simulink model "design_top"  (R2014a)
settings: Solver=ode45  StartTime=0.0  StopTime=10.0  RelTol=1e-3
settings Model: Creator=jan  LastModifiedBy=jan

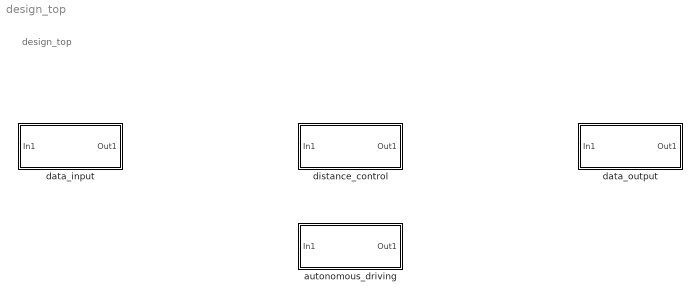
== system design_top ==
  note: design_top
  autonomous_driving : Subsystem
  data_input : Subsystem
  data_output : Subsystem
  distance_control : Subsystem

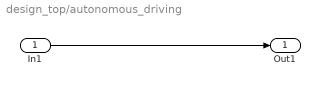
== system design_top/autonomous_driving ==
  In1 : Inport
  Out1 : Outport
  wires:
  In1/1 -> Out1/1

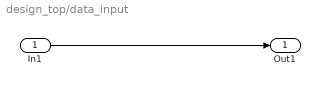
== system design_top/data_input ==
  In1 : Inport
  Out1 : Outport
  wires:
  In1/1 -> Out1/1

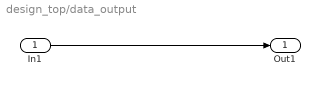
== system design_top/data_output ==
  In1 : Inport
  Out1 : Outport
  wires:
  In1/1 -> Out1/1

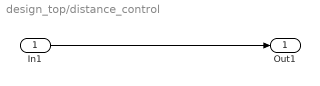
== system design_top/distance_control ==
  In1 : Inport
  Out1 : Outport
  wires:
  In1/1 -> Out1/1
